simulink model "module10"  (R2013a)
settings: Solver=ode3  StartTime=0.0  StopTime=0.5  FixedStep=Ts/10  RelTol=1e-3
InitFcn:
  | Fs = 100;
  | Ts = 1/Fs;
undefined symbols (not defined in the file or in its folder): dfilt
libraries: dsparch4 x1
settings Model: Creator=Lee  LastModifiedBy=cory

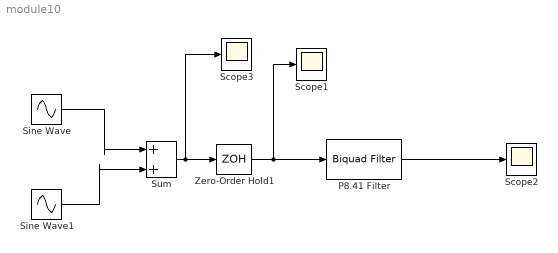
== system module10 ==
  P8.41 Filter : dsparch4/Biquad Filter  Tag=BlockMethodSubSystem  IIRFiltStruct=Direct form II  CoeffSource=Specify via dialog  BiQuadCoeffs=[1 0.030615271301069648 1 1 -0.40554269106751673 0.80989535401212154;1 0.28571428571428514 1 1 -0.22803648852816497 0.50303483764339085;1 0.83050395098945462 1 1 -0.012988613264674738 0.25706873416682885;1 1.5810918329858568 1 1 0.17262553505918118 0.081385259503934368;1 1 0 1 0.1238769766736436 0]  a0Flag=Warning  IC=0  ICnum=0  ICden=0  InputProcessing=Columns as channels (frame based)  denAccumFracLength=30  denProdOutputFracLength=30  secondMemoryFracLength=15  roundingMode=Floor  overflowMode=off  ScaleValues=[0.69158972789798756;0.55781177773791146;0.43952601460501861;0.35017554786288219;0.56193848833682181;1]  optimizeScaleValues=on  ScaleValueMode=Specify via input port (g)  scaleValueFracLength=14  FilterSource=Specify via dialog  dfiltObjectName=dfilt.df2tsos([1 0.3 0.4],[1 0.1 0.2])
  Scope1 : Scope
      settings: TimeRange=0.09052471482889736  YMin=-0.90625  YMax=1.15625
  Scope2 : Scope
      settings: TimeRange=0.09052471482889736  YMin=-0.90625  YMax=1.15625
  Scope3 : Scope
      settings: TimeRange=0.09052471482889736  YMin=-0.90625  YMax=1.15625  SaveName=ScopeData2
  Sine Wave : Sin  Amplitude=3  Frequency=40*pi  SampleTime=0
  Sine Wave1 : Sin  Amplitude=3  Frequency=50*pi  Phase=pi/2  SampleTime=0
  Sum : Sum  Inputs=|++|
  Zero-Order Hold1 : ZeroOrderHold  SampleTime=Ts
  wires:
  Sine Wave1/1 -> Sum/2
  Sine Wave/1 -> Sum/1
  Sum/1 -> Scope3/1, Zero-Order Hold1/1
  Zero-Order Hold1/1 -> P8.41 Filter/1, Scope1/1
  P8.41 Filter/1 -> Scope2/1
